simulink library "dlbsBlockBias"  (R2025b)
settings: Solver=VariableStepAuto  StartTime=0.0  StopTime=10.0  RelTol=1e-3
libraries: dlbsBlockExtractGradientGF x1, dlbsBlockInsertGradientGF x1
settings Model: Creator=lt6037  LastModifiedBy=lt6037

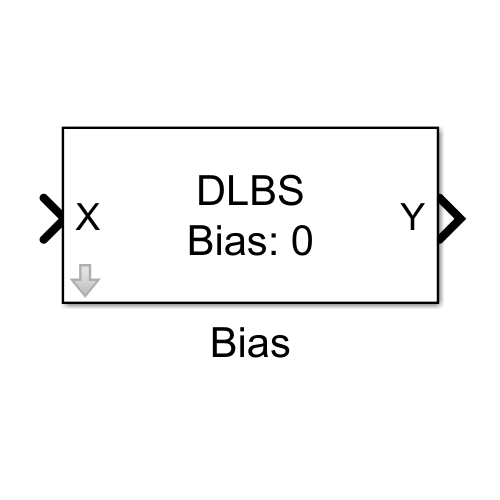
[thumbnail: Simulink's stored preview of the top-level diagram]
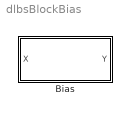
== system dlbsBlockBias ==
  Bias : Subsystem  mask{Bias=0}
      mask prompts: Bias "Simulink:blkprm_prompts:BiasBias"
      mask help: Adds a bias parameter to the input tensor. The operation is applied element-wise across all tensor elements.
      mask Help: web("dlbsHelpBlockBias.html")
      mask TypeOptions Bias: Bias/Bias
      mask DialogControl Bias Prompt: Bias:
      mask Display: fprintf("DLBS\nBias: %s",get(gcbh).Bias)

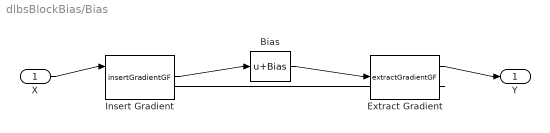
== system dlbsBlockBias/Bias ==
  X : Inport
  Bias : Bias  Bias=Bias  SaturateOnIntegerOverflow=off
  Extract Gradient : dlbsBlockExtractGradientGF/extractGradientGF
  Insert Gradient : dlbsBlockInsertGradientGF/insertGradientGF
  Y : Outport
  wires:
  Extract Gradient/2 -> Insert Gradient/2
  Insert Gradient/1 -> Bias/1
  Bias/1 -> Extract Gradient/1
  Extract Gradient/1 -> Y/1
  X/1 -> Insert Gradient/1
